simulink model "flyback"  (R2023b)
settings: Solver=FixedStepAuto  StartTime=0.0  StopTime=1  FixedStep=1e-6  RelTol=1e-3
model workspace (MAT data in the model file):
  d = 5
  period = 10
  x = 1
values from neighbouring files (symbols this model uses):
  C = Vo-d/(delta_Vc*R*fsw)    [flyback_script.m]
  fsw = 50e3    (= 50000)    [flyback_script.m]
  Lm = abs(Vin*d/(delta_iL*fsw))    [flyback_script.m]
  n = 1/5    (= 0.2)    [flyback_script.m]
  R = Vo^2/Po    (= 7.2)    [flyback_script.m]
  Vin = 100    [flyback_script.m]
libraries: spsCurrentMeasurementLib x7, spsSeriesRLCBranchLib x3, spsVoltageMeasurementLib x3, spsDCVoltageSourceLib x1, spsDiodeLib x1, spsMosfetLib x1, spsVariableRatioTransformerLib x1, sps_lib x1
settings Model: ParameterArgumentNames=x  Creator=ahmeterenlacinbala  LastModifiedBy=ahmeterenlacinbala

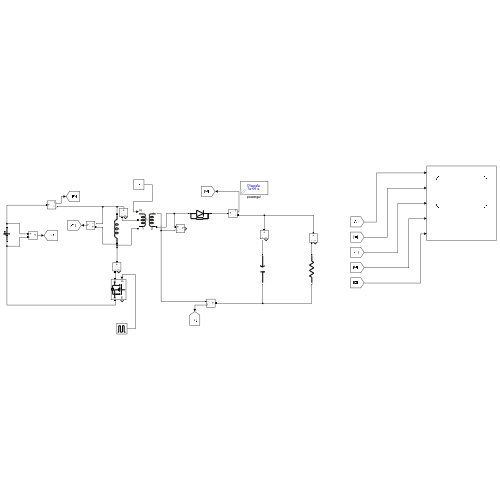
[thumbnail: Simulink's stored preview of the top-level diagram]
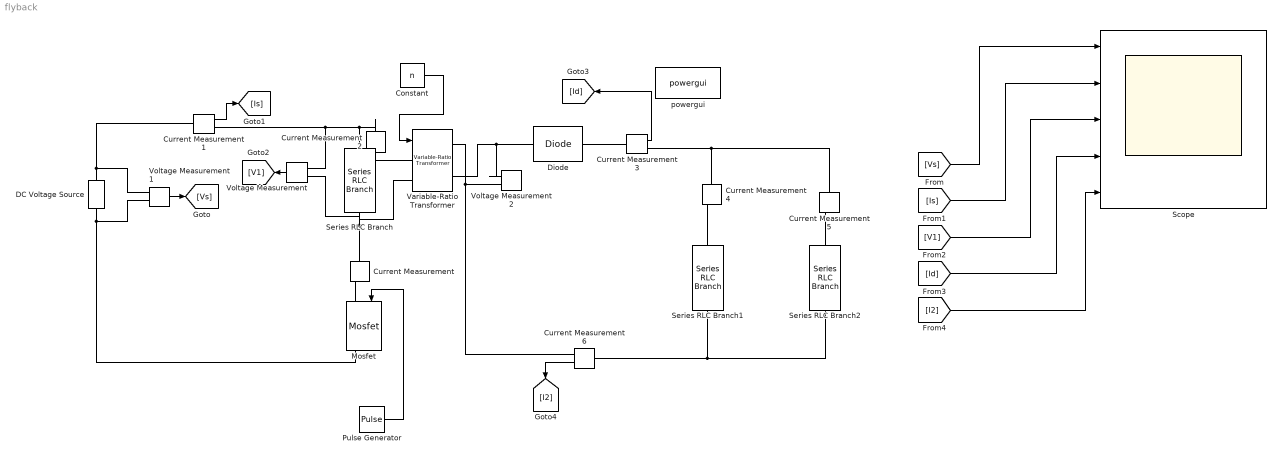
== system flyback ==
  Constant : Constant  Value=n
  Current Measurement{,1..6} (7 alike) : spsCurrentMeasurementLib/Current Measurement  PhasorSimulation=off  OutputType=Complex  PSBequivalent=0
  DC Voltage Source : spsDCVoltageSourceLib/DC Voltage Source  Amplitude=Vin  Measurements=None
  Diode : spsDiodeLib/Diode  Ron=0.001  Lon=0  Vf=0.8  IC=0  UseSnubber=0  Rs=500  Cs=250e-9  Measurements=off
  Mosfet : spsMosfetLib/Mosfet  Ron=0.1  Lon=0  Rd=0.01  Vfd=0  IC=0  Rs=1e5  Cs=inf  Measurements=on
  Pulse Generator : DiscretePulseGenerator  PulseType=Time based  Period=1/fsw  PulseWidth=5
  Scope : Scope  NumInputPorts=5
  Series RLC Branch : spsSeriesRLCBranchLib/Series RLC Branch  LConnTagsString=__new0  RConnTagsString=__new0  BranchType=L  Resistance=1  Inductance=Lm  SetiL0=off  InitialCurrent=0  Capacitance=1e-6  Setx0=off  InitialVoltage=0  Measurements=None
  Series RLC Branch1 : spsSeriesRLCBranchLib/Series RLC Branch  LConnTagsString=__new0  RConnTagsString=__new0  BranchType=C  Resistance=1  Inductance=145e-3  SetiL0=off  InitialCurrent=0  Capacitance=C  Setx0=off  InitialVoltage=0  Measurements=None
  Series RLC Branch2 : spsSeriesRLCBranchLib/Series RLC Branch  LConnTagsString=__new0  RConnTagsString=__new0  BranchType=R  Resistance=R  Inductance=145e-3  SetiL0=off  InitialCurrent=0  Capacitance=1e-6  Setx0=off  InitialVoltage=0  Measurements=None
  Variable-Ratio Transformer : spsVariableRatioTransformerLib/Variable-Ratio Transformer
      settings: LibrarySourceBlock=|
      | sps_lib/Passives/Variable-Ratio
      | Transformer
  Voltage Measurement : spsVoltageMeasurementLib/Voltage Measurement  PhasorSimulation=off  OutputType=Complex  PSBequivalent=0
  Voltage Measurement1 : spsVoltageMeasurementLib/Voltage Measurement  PhasorSimulation=off  OutputType=Complex  PSBequivalent=0
  Voltage Measurement2 : spsVoltageMeasurementLib/Voltage Measurement  PhasorSimulation=off  OutputType=Complex  PSBequivalent=0
  powergui : sps_lib/powergui  Priority=1  SimulationMode=Discrete  SampleTime=1e-6  frequency=60  Iterations=50  frequencyindice=0  Pbase=100e6  ErrMax=1e-4  UnitsV=kV  UnitsW=MW  buscounter=0  FunctionMessages=off  echomessages=off  EnableUseOfTLC=off  CurrentSourceSwitches=off  DisableSnubberDevices=off  DisableRonSwitches=off  DisableVfSwitches=off  DisplayEquations=off  AutomaticDiscreteSolvers=off  SolverType=Tustin/Backward Euler (TBE)  Interpol=off  ExternalGateDelay=off  methode=off  Ts=100  x0status=blocks  SPID=on  SwTol=0  HookPort=off  NonlinearTolerance=1e-4  nMaxIteration=100  ContinueOnMaxIteration=off  RestoreLinks=warning  ResistiveCurrentMeasurement=off  Frange=[0:2:500]  Ylog=off  Xlog=on  ShowGrid=off  save=off  variable=ZData  structure=0  ZoomFFT=off  StartTime=0.0  cycles=1  DisplayStyle=1  fundamental=60  FreqAxis=off  MaxFrequency=1000  frequencyindicesteady=1  RmsSteady=1  display=off
  wires:
  Voltage Measurement1/1 -> [Vs]
  Current Measurement1/1 -> [Is]
  Voltage Measurement/1 -> [V1]
  Current Measurement3/1 -> [Id]
  Current Measurement6/1 -> [I2]
  Constant/1 -> Variable-Ratio Transformer/1
  [Vs] -> Scope/1
  [Is] -> Scope/2
  [V1] -> Scope/3
  [Id] -> Scope/4
  [I2] -> Scope/5
  Pulse Generator/1 -> Mosfet/1
  connections:
  Voltage Measurement/LConn2 -- Series RLC Branch/RConn1 -- Current Measurement2/LConn1 -- Current Measurement1/RConn1
  DC Voltage Source/LConn1 -- Voltage Measurement1/LConn2 -- Mosfet/RConn1
  Series RLC Branch/LConn1 -- Variable-Ratio Transformer/LConn2 -- Voltage Measurement/LConn1 -- Current Measurement/LConn1
  Current Measurement/RConn1 -- Mosfet/LConn1
  DC Voltage Source/RConn1 -- Voltage Measurement1/LConn1 -- Current Measurement1/LConn1
  Current Measurement2/RConn1 -- Variable-Ratio Transformer/LConn1
  Voltage Measurement2/LConn1 -- Diode/LConn1 -- Variable-Ratio Transformer/RConn2
  Current Measurement3/LConn1 -- Diode/RConn1
  Current Measurement3/RConn1 -- Current Measurement4/LConn1 -- Current Measurement5/LConn1
  Series RLC Branch1/RConn1 -- Current Measurement4/RConn1
  Series RLC Branch1/LConn1 -- Current Measurement6/LConn1 -- Series RLC Branch2/LConn1
  Current Measurement5/RConn1 -- Series RLC Branch2/RConn1
  Voltage Measurement2/LConn2 -- Current Measurement6/RConn1 -- Variable-Ratio Transformer/RConn1
